simulink model "HA3_model_instr"  (R2013b)
settings: Solver=ode45  StartTime=0.0  StopTime=10.0  RelTol=1e-3
settings Model: Creator=adokhanc  LastModifiedBy=georgios
settings DataIOCC: SaveFormat=StructureWithTime
settings DebuggingCC: FrameProcessingCompatibilityMsg=error  StateNameClashWarn=warning
settings GRTTargetCC: CodeReplacementLibrary=C89/C90 (ANSI)

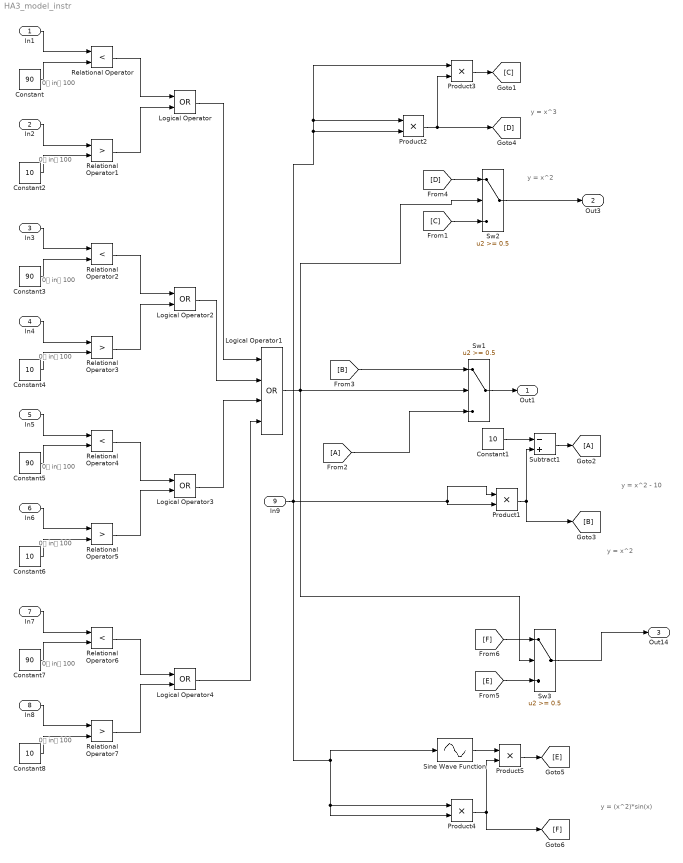
== system HA3_model_instr ==
  note: 0 in 100
  note: 0 in 100
  note: 0 in 100
  note: 0 in 100
  note: 0 in 100
  note: 0 in 100
  note: 0 in 100
  note: 0 in 100
  note: y = x^2
  note: y = x^2 - 10
  note: y = x^2
  note: y = x^3
  note: y = (x^2)*sin(x)
  In1 : Inport
  In2 : Inport  Port=2
  In3 : Inport  Port=3
  In4 : Inport  Port=4
  In5 : Inport  Port=5
  In6 : Inport  Port=6
  In7 : Inport  Port=7
  In8 : Inport  Port=8
  In9 : Inport  Port=9  OutDataTypeStr=double
  Constant{,3,5,7} (4 alike) : Constant  Value=90
  Constant1 : Constant  Value=10  OutDataTypeStr=Inherit: Inherit via back propagation
  Constant{2,4,6,8} (4 alike) : Constant  Value=10
  Logical Operator{,2..4} (4 alike) : Logic  Operator=OR  AllPortsSameDT=off  OutDataTypeStr=boolean
  Logical Operator1 : Logic  Operator=OR  Inputs=4  AllPortsSameDT=off  OutDataTypeStr=boolean
  Product1 : Product  OutDataTypeStr=double  RndMeth=Zero
  Product{2..5} (4 alike) : Product  RndMeth=Zero
  Relational Operator{,2,4,6} (4 alike) : RelationalOperator  Operator=<  OutDataTypeStr=boolean
  Relational Operator{1,3,5,7} (4 alike) : RelationalOperator  Operator=>  OutDataTypeStr=boolean
  Sine Wave Function : Sin  TimeSource=Use external signal  SampleTime=0
  Subtract1 : Sum  Inputs=-+
  Sw1 : Switch  Threshold=0.5  OutDataTypeStr=double  RndMeth=Simplest  InputSameDT=on
  Sw2 : Switch  Threshold=0.5  RndMeth=Simplest  InputSameDT=on
  Sw3 : Switch  Threshold=0.5  RndMeth=Simplest  InputSameDT=on
  Out1 : Outport
  Out3 : Outport  Port=2
  Out14 : Outport  Port=3
  wires:
  Product1/1 -> Subtract1/2, [B]
  Constant1/1 -> Subtract1/1
  Subtract1/1 -> [A]
  Constant/1 -> Relational Operator/2
  Constant2/1 -> Relational Operator1/2
  Relational Operator/1 -> Logical Operator/1
  Relational Operator1/1 -> Logical Operator/2
  Constant3/1 -> Relational Operator2/2
  Constant4/1 -> Relational Operator3/2
  Relational Operator2/1 -> Logical Operator2/1
  Relational Operator3/1 -> Logical Operator2/2
  Constant5/1 -> Relational Operator4/2
  Constant6/1 -> Relational Operator5/2
  Relational Operator4/1 -> Logical Operator3/1
  Relational Operator5/1 -> Logical Operator3/2
  Constant7/1 -> Relational Operator6/2
  Constant8/1 -> Relational Operator7/2
  Relational Operator6/1 -> Logical Operator4/1
  Relational Operator7/1 -> Logical Operator4/2
  Logical Operator/1 -> Logical Operator1/1
  Logical Operator2/1 -> Logical Operator1/2
  Logical Operator3/1 -> Logical Operator1/3
  Product2/1 -> [D], Product3/2
  Product3/1 -> [C]
  [D] -> Sw2/1
  [C] -> Sw2/3
  [F] -> Sw3/1
  [E] -> Sw3/3
  Product4/1 -> [F], Product5/2
  Product5/1 -> [E]
  Sine Wave Function/1 -> Product5/1
  In1/1 -> Relational Operator/1
  In2/1 -> Relational Operator1/1
  In3/1 -> Relational Operator2/1
  In4/1 -> Relational Operator3/1
  In5/1 -> Relational Operator4/1
  In6/1 -> Relational Operator5/1
  In7/1 -> Relational Operator6/1
  In8/1 -> Relational Operator7/1
  Logical Operator1/1 -> Sw1/2, Sw3/2, Sw2/2
  Sw3/1 -> Out14/1
  Sw2/1 -> Out3/1
  Sw1/1 -> Out1/1
  [B] -> Sw1/1
  In9/1 -> Product4/1, Product4/2, Sine Wave Function/1, Product2/1, Product3/1, Product2/2, Product1/2, Product1/1
  [A] -> Sw1/3
  Logical Operator4/1 -> Logical Operator1/4
